simulink model "planar_quad_animation"  (R2015a)
settings: Solver=ode45  StartTime=0.0  StopTime=inf  RelTol=1e-3
undefined symbols (not defined in the file or in its folder): drawPlanarQuad
libraries: simulink x2
settings Model: Creator=ecestudent  LastModifiedBy=ecestudent

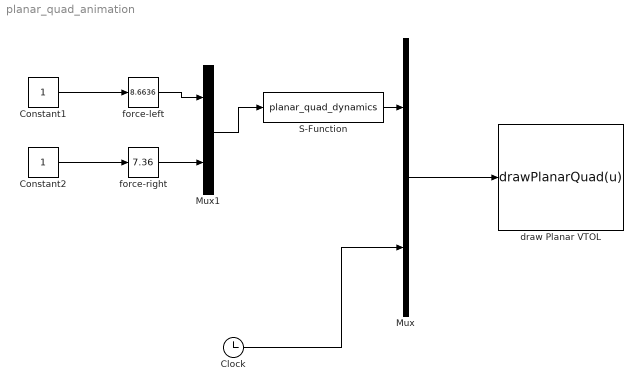
== system planar_quad_animation ==
  Clock : Clock
  Constant1 : Constant
  Constant2 : Constant
  Mux : Mux  Inputs=2
  Mux1 : Mux  Inputs=2
  S-Function : S-Function  FunctionName=planar_quad_dynamics  Parameters=AP
  draw Planar VTOL : MATLABFcn  MATLABFcn=drawPlanarQuad(u)  OutputDimensions=0
      mask Display: image(imread('tv.jpg'))
  force-left : simulink/Math Operations/Slider Gain  low=0  gain=8.6636  high=10
  force-right : simulink/Math Operations/Slider Gain  low=0  gain=7.36  high=10
  wires:
  Constant1/1 -> force-left/1
  Constant2/1 -> force-right/1
  Clock/1 -> Mux/2
  Mux/1 -> draw Planar VTOL/1
  force-right/1 -> Mux1/2
  force-left/1 -> Mux1/1
  S-Function/1 -> Mux/1
  Mux1/1 -> S-Function/1
